simulink model "Stewart_simple"  (R2014a)
settings: Solver=ode3  SolverMode=SingleTasking  StartTime=0.0  StopTime=inf  RelTol=1e-3
libraries: arduinolib x18, neural x6, simulink x1
settings Model: SimulationMode=external  CovModelRefEnable=off  CovSFcnEnable=on  ExtModeTrigDuration=2  Creator=costa  LastModifiedBy=rcostado
settings OptimizationCC: OptimizeModelRefInitCode=on  LifeSpan=1
settings DebuggingCC: UnderspecifiedInitializationDetection=Classic  SolverPrmCheckMsg=none
settings HardwareCC: ProdBitPerInt=16  ProdBitPerPointer=8  ProdIntDivRoundTo=Zero  ProdEndianess=LittleEndian  ProdWordSize=8  ProdHWDeviceType=Atmel->AVR
settings RTWCC: SystemTargetFile=realtime.tlc  GenerateMakefile=off  TemplateMakefile=realtime.tmf  Description=Run on Target Hardware  RTWVerbose=off  ProcessScript=realtime_make_rtw_hook
settings STFCustomTargetCC: TargetLibSuffix=.a  GenerateSampleERTMain=on  ConcurrentExecutionCompliant=off  GeneratePreprocessorConditionals=Use local settings  ERTCustomFileBanners=on  SupportNonInlinedSFcns=off  SupportVariableSizeSignals=on  MATLABClassNameForMDSCustomization=Simulink.SoftwareTarget.ERTCustomization  GRTInterface=off  SystemTargetFile=realtime.tlc
settings ERTTargetCC: CombineOutputUpdateFcns=off  SupportContinuousTime=on  SupportVariableSizeSignals=on  ExtModeTransport=3  ExtModeMexFile=ext_serial_win32_comm  ExtModeMexArgs=0 1 9600  ERTSrcFileBannerTemplate=realtime_code_template.cgt  ERTHdrFileBannerTemplate=realtime_code_template.cgt  ERTDataSrcFileTemplate=realtime_code_template.cgt  ERTDataHdrFileTemplate=realtime_code_template.cgt  ERTCustomFileTemplate=realtime_file_process.tlc

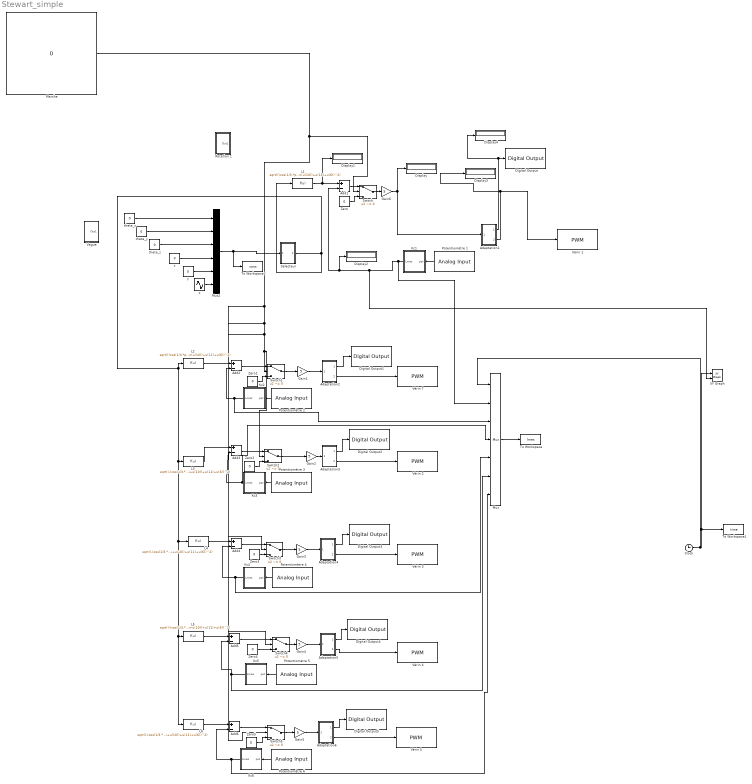
== system Stewart_simple ==
  Adaptation1 : Subsystem
  Adaptation2 : Subsystem
  Adaptation3 : Subsystem
  Adaptation4 : Subsystem
  Adaptation5 : Subsystem
  Adaptation6 : Subsystem
  Add{1..6} (6 alike) : Sum  Inputs=+-
  Clock : Clock
  Digital Output : arduinolib/Digital Output  pinNumber=11
  Digital Output1 : arduinolib/Digital Output  pinNumber=5
  Digital Output2 : arduinolib/Digital Output  pinNumber=3
  Digital Output3 : arduinolib/Digital Output  pinNumber=9
  Digital Output4 : arduinolib/Digital Output  pinNumber=7
  Digital Output5 : arduinolib/Digital Output  pinNumber=13
  Display{,1..4} (5 alike) : Display
  Gain{1..6} (6 alike) : Gain  Gain=5
  Kc1 : Subsystem
  Kc2 : Subsystem
  Kc3 : Subsystem
  Kc4 : Subsystem
  Kc5 : Subsystem
  Kc6 : Subsystem
  L1 : Fcn  Expr=sqrt(((cos(1/3.*pi+u(3))*cos(u(2))-sin(1/3.*pi+u(3))*sin(u(1))*sin(u(2)))*u(7)*cos(u(10))+sin(1/3.*pi+u(3))*cos(u(1))*u(7)*sin(u(10))-u(8)*cos(u(9))+u(4))^2+ ((sin(1/3.*pi+u(3))*cos(u(2))+cos(1/3.*pi+u(3))*sin(u(1))*sin(u(2)))*u(7)*cos(u(10))-cos(1/3.*pi+u(3))*cos(u(1))*u(7)*sin(u(10))-u(8)*sin(u(9))+u(5))^2+ (-cos(u(1))*sin(u(2))*u(7)*cos(u(10))-sin(u(1))*u(7)*sin(u(10))+u(11)+u(6))^2)
  L2 : Fcn  Expr=sqrt(((cos(1/3.*pi+u(3))*cos(u(2))-sin(1/3.*pi+u(3))*sin(u(1))*sin(u(2)))*u(7)*cos(u(10))-sin(1/3.*pi+u(3))*cos(u(1))*u(7)*sin(u(10))+u(8)*cos(1/3.*pi+u(9))+u(4))^2+ ((sin(1/3.*pi+u(3))*cos(u(2))+cos(1/3.*pi+u(3))*sin(u(1))*sin(u(2)))*u(7)*cos(u(10))+cos(1/3.*pi+u(3))*cos(u(1))*u(7)*sin(u(10))-u(8)*sin(1/3.*pi+u(9))+u(5))^2+ (-cos(u(1))*sin(u(2))*u(7)*cos(u(10))+sin(u(1))*u(7)*sin(u(10))+u(11)+u(6))^2)
  L3 : Fcn  Expr=sqrt((-(cos(1/3.*pi+u(3))*cos(u(2))-sin(1/3.*pi+u(3))*sin(u(1))*sin(u(2)))*u(7)*cos(1/3.*pi+u(10))-sin(1/3.*pi+u(3))*cos(u(1))*u(7)*sin(1/3.*pi+u(10))+u(8)*sin(1/6.*pi+u(9))+u(4))^2+(-(sin(1/3.*pi+u(3))*cos(u(2))+cos(1/3.*pi+u(3))*sin(u(1))*sin(u(2)))*u(7)*cos(1/3.*pi+u(10))+cos(1/3.*pi+u(3))*cos(u(1))*u(7)*sin(1/3.*pi+u(10))-u(8)*cos(1/6.*pi+u(9))+u(5))^2+(cos(u(1))*sin(u(2))*u(7)*cos(1/3.*pi+u(10))+sin(u(1))*u(7)*sin(1/3.*pi+u(10))+u(11)+u(6))^2)
  L4 : Fcn  Expr=sqrt((-(cos(1/3.*pi+u(3))*cos(u(2))-sin(1/3.*pi+u(3))*sin(u(1))*sin(u(2)))*u(7)*sin(1/6.*pi+u(10))-sin(1/3.*pi+u(3))*cos(u(1))*u(7)*cos(1/6.*pi+u(10))+u(8)*sin(1/6.*pi+u(9))+u(4))^2+(-(sin(1/3.*pi+u(3))*cos(u(2))+cos(1/3.*pi+u(3))*sin(u(1))*sin(u(2)))*u(7)*sin(1/6.*pi+u(10))+cos(1/3.*pi+u(3))*cos(u(1))*u(7)*cos(1/6.*pi+u(10))+u(8)*cos(1/6.*pi+u(9))+u(5))^2+(cos(u(1))*sin(u(2))*u(7)*sin(1/6.*pi+u(10))+sin(u(1))*u(7)*cos(1/6.*pi+u(10))+u(11)+u(6))^2)
  L5 : Fcn  Expr=sqrt((-(cos(1/3.*pi+u(3))*cos(u(2))-sin(1/3.*pi+u(3))*sin(u(1))*sin(u(2)))*u(7)*sin(1/6.*pi+u(10))+sin(1/3.*pi+u(3))*cos(u(1))*u(7)*cos(1/6.*pi+u(10))+u(8)*cos(1/3.*pi+u(9))+u(4))^2+(-(sin(1/3.*pi+u(3))*cos(u(2))+cos(1/3.*pi+u(3))*sin(u(1))*sin(u(2)))*u(7)*sin(1/6.*pi+u(10))-cos(1/3.*pi+u(3))*cos(u(1))*u(7)*cos(1/6.*pi+u(10))+u(8)*sin(1/3.*pi+u(9))+u(5))^2+(cos(u(1))*sin(u(2))*u(7)*sin(1/6.*pi+u(10))-sin(u(1))*u(7)*cos(1/6.*pi+u(10))+u(11)+u(6))^2)
  L6 : Fcn  Expr=sqrt((-(cos(1/3.*pi+u(3))*cos(u(2))-sin(1/3.*pi+u(3))*sin(u(1))*sin(u(2)))*u(7)*cos(1/3.*pi+u(10))+sin(1/3.*pi+u(3))*cos(u(1))*u(7)*sin(1/3.*pi+u(10))-u(8)*cos(u(9))+u(4))^2+(-(sin(1/3.*pi+u(3))*cos(u(2))+cos(1/3.*pi+u(3))*sin(u(1))*sin(u(2)))*u(7)*cos(1/3.*pi+u(10))-cos(1/3.*pi+u(3))*cos(u(1))*u(7)*sin(1/3.*pi+u(10))+u(8)*sin(u(9))+u(5))^2+(cos(u(1))*sin(u(2))*u(7)*cos(1/3.*pi+u(10))-sin(u(1))*u(7)*sin(1/3.*pi+u(10))+u(11)+u(6))^2)
  Marche : Constant  Value=0
  Mux : Mux  Inputs=7
  Mux2 : Mux  Inputs=6
  Potentiomètre 1 : arduinolib/Analog Input  pinNumber=2  sampleTime=0.001
  Potentiomètre 2 : arduinolib/Analog Input  pinNumber=1  sampleTime=0.001
  Potentiomètre 3 : arduinolib/Analog Input  pinNumber=0  sampleTime=0.001
  Potentiomètre 4 : arduinolib/Analog Input  pinNumber=5  sampleTime=0.001
  Potentiomètre 5 : arduinolib/Analog Input  pinNumber=4  sampleTime=0.001
  Potentiomètre 6 : arduinolib/Analog Input  pinNumber=3  sampleTime=0.001
  Rotation z : Subsystem
  Selecteur : Subsystem
  Switch{,1..5} (6 alike) : Switch  Criteria=u2 ~= 0
  To Workspace : ToWorkspace  VariableName=lmes  SampleTime=-1
  To Workspace1 : ToWorkspace  VariableName=time  SampleTime=-1
  To Workspace2 : ToWorkspace  VariableName=cons  SampleTime=-1
  Vague : Subsystem
  Vérin 1 : arduinolib/PWM  pinNumber=10
  Vérin 2 : arduinolib/PWM  pinNumber=2
  Vérin 3 : arduinolib/PWM  pinNumber=8
  Vérin 4 : arduinolib/PWM  pinNumber=6
  Vérin 5 : arduinolib/PWM  pinNumber=12
  Vérin 7 : arduinolib/PWM  pinNumber=4
  XY Graph : simulink/Sinks/XY Graph  xmin=0  xmax=10  ymin=300  ymax=600  st=-1
  Zero{,1..5} (6 alike) : Constant  Value=0
  theta_x : Constant  Value=0
  theta_y : Constant  Value=0
  theta_z : Constant  Value=0
  x : Constant  Value=0
  y : Constant  Value=0
  z : Sin  Amplitude=50  Frequency=60  SampleTime=0
  wires:
  Potentiomètre 1/1 -> Kc1/1(pot)
  L1/1 -> Display1/1, Add1/1
  Gain6/1 -> Display/1, Adaptation1/1(ecart)
  Adaptation1/1(sens) -> Display4/1, Digital Output/1
  Adaptation1/2(pwm) -> Display3/1, Vérin 1/1
  Selecteur/1(Out1) -> L6/1, L5/1, L4/1, L3/1, L2/1, L1/1
  Mux2/1 -> To Workspace2/1, Selecteur/1(In2)
  Gain1/1 -> Adaptation2/1(ecart)
  L2/1 -> Add2/1
  Adaptation2/1(sens) -> Digital Output1/1
  Adaptation2/2(pwm) -> Vérin 7/1
  Potentiomètre 2/1 -> Kc2/1(pot)
  Kc2/1(Lmes) -> Mux/3, Add2/2
  L3/1 -> Add3/1
  Adaptation3/1(sens) -> Digital Output2/1
  Adaptation3/2(pwm) -> Vérin 2/1
  Gain2/1 -> Adaptation3/1(ecart)
  Potentiomètre 3/1 -> Kc3/1(pot)
  L4/1 -> Add4/1
  Gain3/1 -> Adaptation4/1(ecart)
  Adaptation4/1(sens) -> Digital Output3/1
  Adaptation4/2(pwm) -> Vérin 3/1
  Kc4/1(Lmes) -> Mux/5, Add4/2
  Potentiomètre 4/1 -> Kc4/1(pot)
  L5/1 -> Add5/1
  Adaptation5/1(sens1) -> Digital Output4/1
  Adaptation5/2(pwm1) -> Vérin 4/1
  Potentiomètre 5/1 -> Kc5/1(pot)
  Kc5/1(Lmes) -> Mux/6, Add5/2
  Gain4/1 -> Adaptation5/1(ecart1)
  L6/1 -> Add6/1
  Adaptation6/1(sens) -> Digital Output5/1
  Adaptation6/2(pwm) -> Vérin 5/1
  Potentiomètre 6/1 -> Kc6/1(pot)
  Kc6/1(Lmes) -> Mux/7, Add6/2
  Gain5/1 -> Adaptation6/1(ecart)
  Kc1/1(Lmes) -> Mux/2, XY Graph/2, Display2/1, Add1/2
  Kc3/1(Lmes) -> Mux/4, Add3/2
  z/1 -> Mux2/6
  x/1 -> Mux2/4
  theta_x/1 -> Mux2/1
  y/1 -> Mux2/5
  theta_z/1 -> Mux2/3
  theta_y/1 -> Mux2/2
  Switch/1 -> Gain6/1
  Add1/1 -> Switch/1
  Zero/1 -> Switch/3
  Marche/1 -> Switch5/2, Switch3/2, Switch4/2, Switch2/2, Switch1/2, Switch/2
  Add2/1 -> Switch1/1
  Switch1/1 -> Gain1/1
  Zero1/1 -> Switch1/3
  Switch2/1 -> Gain2/1
  Zero2/1 -> Switch2/3
  Zero3/1 -> Switch3/3
  Switch3/1 -> Gain3/1
  Add4/1 -> Switch3/1
  Switch4/1 -> Gain4/1
  Add5/1 -> Switch4/1
  Zero4/1 -> Switch4/3
  Switch5/1 -> Gain5/1
  Zero5/1 -> Switch5/3
  Add6/1 -> Switch5/1
  Add3/1 -> Switch2/1
  Mux/1 -> To Workspace/1
  Clock/1 -> Mux/1, To Workspace1/1, XY Graph/1

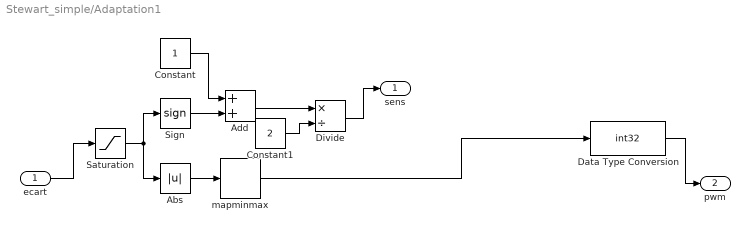
== system Stewart_simple/Adaptation1 ==
  ecart : Inport
  Abs : Abs
  Add : Sum
  Constant : Constant
  Constant1 : Constant  Value=2
  Data Type Conversion : DataTypeConversion  OutDataTypeStr=int32
  Divide : Product  Inputs=*/
  Saturation : Saturate  UpperLimit=200  LowerLimit=-200
  Sign : Signum
  mapminmax : neural/Processing Functions/mapminmax  xmin=0  xmax=200  ymin=1  ymax=255
  sens : Outport
  pwm : Outport  Port=2
  wires:
  ecart/1 -> Saturation/1
  Abs/1 -> mapminmax/1
  Saturation/1 -> Sign/1, Abs/1
  Sign/1 -> Add/2
  Constant/1 -> Add/1
  Add/1 -> Divide/1
  Constant1/1 -> Divide/2
  Divide/1 -> sens/1
  Data Type Conversion/1 -> pwm/1
  mapminmax/1 -> Data Type Conversion/1

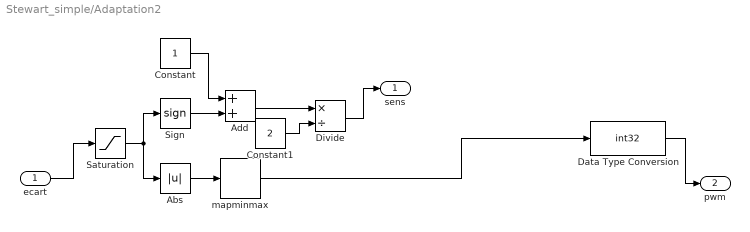
== system Stewart_simple/Adaptation2 ==
  ecart : Inport
  Abs : Abs
  Add : Sum
  Constant : Constant
  Constant1 : Constant  Value=2
  Data Type Conversion : DataTypeConversion  OutDataTypeStr=int32
  Divide : Product  Inputs=*/
  Saturation : Saturate  UpperLimit=200  LowerLimit=-200
  Sign : Signum
  mapminmax : neural/Processing Functions/mapminmax  xmin=0  xmax=200  ymin=1  ymax=255
  sens : Outport
  pwm : Outport  Port=2
  wires:
  ecart/1 -> Saturation/1
  Abs/1 -> mapminmax/1
  Saturation/1 -> Sign/1, Abs/1
  Sign/1 -> Add/2
  Constant/1 -> Add/1
  Add/1 -> Divide/1
  Constant1/1 -> Divide/2
  Divide/1 -> sens/1
  Data Type Conversion/1 -> pwm/1
  mapminmax/1 -> Data Type Conversion/1

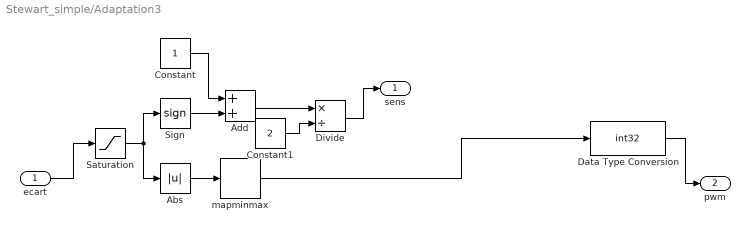
== system Stewart_simple/Adaptation3 ==
  ecart : Inport
  Abs : Abs
  Add : Sum
  Constant : Constant
  Constant1 : Constant  Value=2
  Data Type Conversion : DataTypeConversion  OutDataTypeStr=int32
  Divide : Product  Inputs=*/
  Saturation : Saturate  UpperLimit=200  LowerLimit=-200
  Sign : Signum
  mapminmax : neural/Processing Functions/mapminmax  xmin=0  xmax=200  ymin=1  ymax=255
  sens : Outport
  pwm : Outport  Port=2
  wires:
  ecart/1 -> Saturation/1
  Abs/1 -> mapminmax/1
  Saturation/1 -> Sign/1, Abs/1
  Sign/1 -> Add/2
  Constant/1 -> Add/1
  Add/1 -> Divide/1
  Constant1/1 -> Divide/2
  Divide/1 -> sens/1
  Data Type Conversion/1 -> pwm/1
  mapminmax/1 -> Data Type Conversion/1

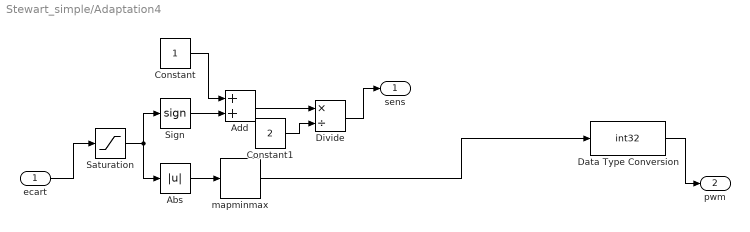
== system Stewart_simple/Adaptation4 ==
  ecart : Inport
  Abs : Abs
  Add : Sum
  Constant : Constant
  Constant1 : Constant  Value=2
  Data Type Conversion : DataTypeConversion  OutDataTypeStr=int32
  Divide : Product  Inputs=*/
  Saturation : Saturate  UpperLimit=200  LowerLimit=-200
  Sign : Signum
  mapminmax : neural/Processing Functions/mapminmax  xmin=0  xmax=200  ymin=1  ymax=255
  sens : Outport
  pwm : Outport  Port=2
  wires:
  ecart/1 -> Saturation/1
  Abs/1 -> mapminmax/1
  Saturation/1 -> Sign/1, Abs/1
  Sign/1 -> Add/2
  Constant/1 -> Add/1
  Add/1 -> Divide/1
  Constant1/1 -> Divide/2
  Divide/1 -> sens/1
  Data Type Conversion/1 -> pwm/1
  mapminmax/1 -> Data Type Conversion/1

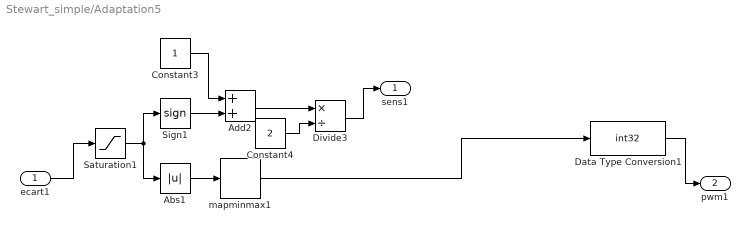
== system Stewart_simple/Adaptation5 ==
  ecart1 : Inport
  Abs1 : Abs
  Add2 : Sum
  Constant3 : Constant
  Constant4 : Constant  Value=2
  Data Type Conversion1 : DataTypeConversion  OutDataTypeStr=int32
  Divide3 : Product  Inputs=*/
  Saturation1 : Saturate  UpperLimit=200  LowerLimit=-200
  Sign1 : Signum
  mapminmax1 : neural/Processing Functions/mapminmax  xmin=0  xmax=200  ymin=1  ymax=255
  sens1 : Outport
  pwm1 : Outport  Port=2
  wires:
  ecart1/1 -> Saturation1/1
  Abs1/1 -> mapminmax1/1
  Saturation1/1 -> Sign1/1, Abs1/1
  Sign1/1 -> Add2/2
  Constant3/1 -> Add2/1
  Add2/1 -> Divide3/1
  Constant4/1 -> Divide3/2
  Divide3/1 -> sens1/1
  Data Type Conversion1/1 -> pwm1/1
  mapminmax1/1 -> Data Type Conversion1/1

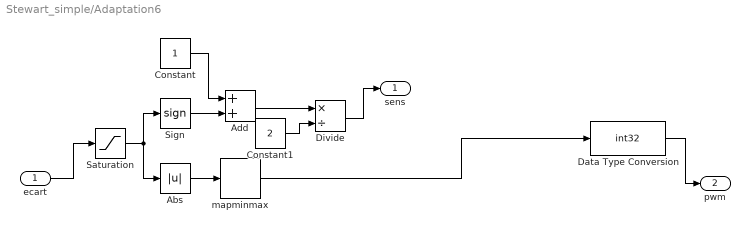
== system Stewart_simple/Adaptation6 ==
  ecart : Inport
  Abs : Abs
  Add : Sum
  Constant : Constant
  Constant1 : Constant  Value=2
  Data Type Conversion : DataTypeConversion  OutDataTypeStr=int32
  Divide : Product  Inputs=*/
  Saturation : Saturate  UpperLimit=200  LowerLimit=-200
  Sign : Signum
  mapminmax : neural/Processing Functions/mapminmax  xmin=0  xmax=200  ymin=1  ymax=255
  sens : Outport
  pwm : Outport  Port=2
  wires:
  ecart/1 -> Saturation/1
  Abs/1 -> mapminmax/1
  Saturation/1 -> Sign/1, Abs/1
  Sign/1 -> Add/2
  Constant/1 -> Add/1
  Add/1 -> Divide/1
  Constant1/1 -> Divide/2
  Divide/1 -> sens/1
  Data Type Conversion/1 -> pwm/1
  mapminmax/1 -> Data Type Conversion/1

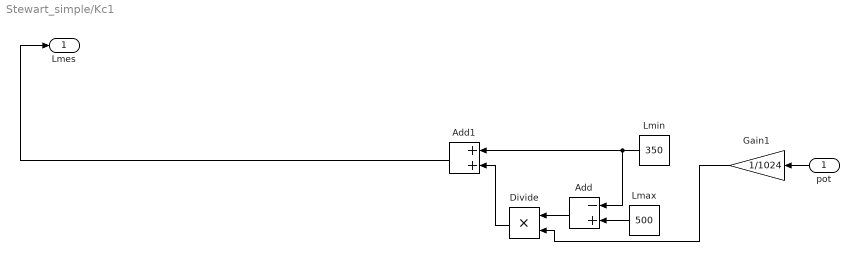
== system Stewart_simple/Kc1 ==
  pot : Inport
  Add : Sum  Inputs=-+
  Add1 : Sum
  Divide : Product  Inputs=**
  Gain1 : Gain  Gain=1/1024
  Lmax : Constant  Value=500
  Lmin : Constant  Value=350
  Lmes : Outport
  wires:
  Lmin/1 -> Add1/1, Add/1
  Lmax/1 -> Add/2
  Gain1/1 -> Divide/2
  Divide/1 -> Add1/2
  Add1/1 -> Lmes/1
  pot/1 -> Gain1/1
  Add/1 -> Divide/1

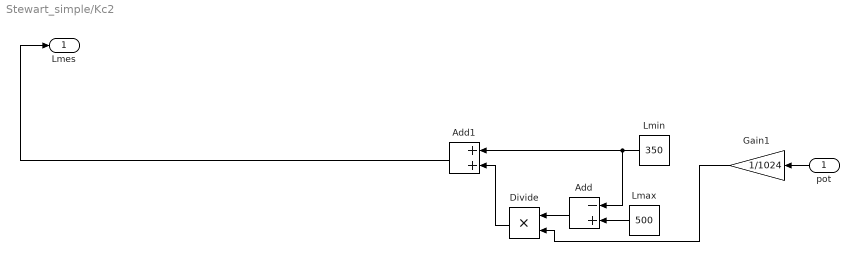
== system Stewart_simple/Kc2 ==
  pot : Inport
  Add : Sum  Inputs=-+
  Add1 : Sum
  Divide : Product  Inputs=**
  Gain1 : Gain  Gain=1/1024
  Lmax : Constant  Value=500
  Lmin : Constant  Value=350
  Lmes : Outport
  wires:
  Lmin/1 -> Add1/1, Add/1
  Lmax/1 -> Add/2
  Gain1/1 -> Divide/2
  Divide/1 -> Add1/2
  Add1/1 -> Lmes/1
  pot/1 -> Gain1/1
  Add/1 -> Divide/1

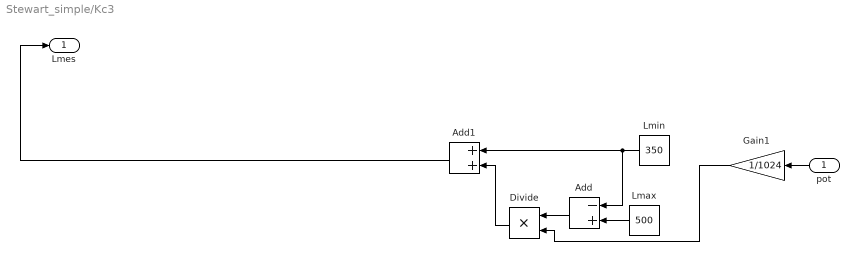
== system Stewart_simple/Kc3 ==
  pot : Inport
  Add : Sum  Inputs=-+
  Add1 : Sum
  Divide : Product  Inputs=**
  Gain1 : Gain  Gain=1/1024
  Lmax : Constant  Value=500
  Lmin : Constant  Value=350
  Lmes : Outport
  wires:
  Lmin/1 -> Add1/1, Add/1
  Lmax/1 -> Add/2
  Gain1/1 -> Divide/2
  Divide/1 -> Add1/2
  Add1/1 -> Lmes/1
  pot/1 -> Gain1/1
  Add/1 -> Divide/1

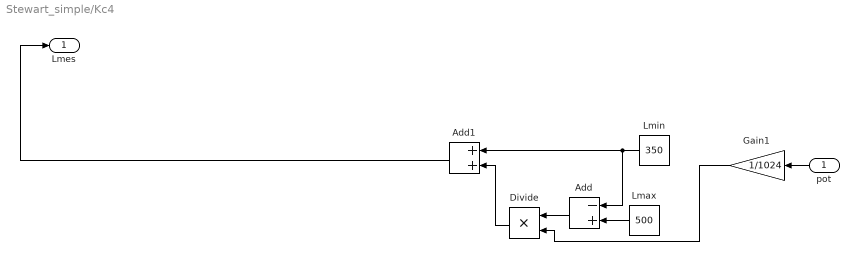
== system Stewart_simple/Kc4 ==
  pot : Inport
  Add : Sum  Inputs=-+
  Add1 : Sum
  Divide : Product  Inputs=**
  Gain1 : Gain  Gain=1/1024
  Lmax : Constant  Value=500
  Lmin : Constant  Value=350
  Lmes : Outport
  wires:
  Lmin/1 -> Add1/1, Add/1
  Lmax/1 -> Add/2
  Gain1/1 -> Divide/2
  Divide/1 -> Add1/2
  Add1/1 -> Lmes/1
  pot/1 -> Gain1/1
  Add/1 -> Divide/1

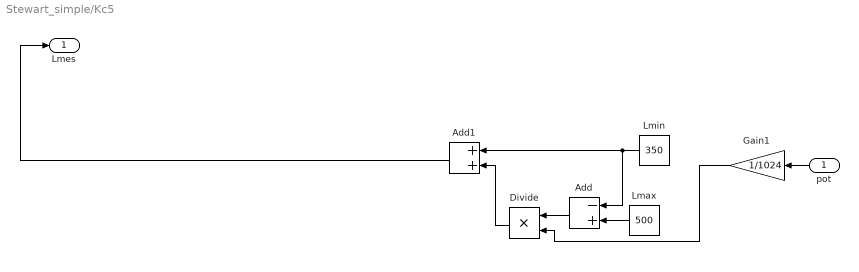
== system Stewart_simple/Kc5 ==
  pot : Inport
  Add : Sum  Inputs=-+
  Add1 : Sum
  Divide : Product  Inputs=**
  Gain1 : Gain  Gain=1/1024
  Lmax : Constant  Value=500
  Lmin : Constant  Value=350
  Lmes : Outport
  wires:
  Lmin/1 -> Add1/1, Add/1
  Lmax/1 -> Add/2
  Gain1/1 -> Divide/2
  Divide/1 -> Add1/2
  Add1/1 -> Lmes/1
  pot/1 -> Gain1/1
  Add/1 -> Divide/1

== system Stewart_simple/Kc6 ==
  pot : Inport
  Add : Sum  Inputs=-+
  Add1 : Sum
  Divide : Product  Inputs=**
  Gain1 : Gain  Gain=1/1024
  Lmax : Constant  Value=500
  Lmin : Constant  Value=350
  Lmes : Outport
  wires:
  Lmin/1 -> Add1/1, Add/1
  Lmax/1 -> Add/2
  Gain1/1 -> Divide/2
  Divide/1 -> Add1/2
  Add1/1 -> Lmes/1
  pot/1 -> Gain1/1
  Add/1 -> Divide/1

== system Stewart_simple/Rotation z ==
  Mux1 : Mux  Inputs=6
  theta_x : Constant  Value=0
  theta_y : Constant  Value=0
  theta_z : Sin  Amplitude=pi/8  Frequency=40  SampleTime=0
  x : Constant  Value=0
  y : Constant  Value=0
  z : Constant  Value=0
  Out1 : Outport
  wires:
  theta_y/1 -> Mux1/2
  theta_z/1 -> Mux1/3
  y/1 -> Mux1/5
  theta_x/1 -> Mux1/1
  x/1 -> Mux1/4
  z/1 -> Mux1/6
  Mux1/1 -> Out1/1

== system Stewart_simple/Selecteur ==
  In2 : Inport
  Mux : Mux  Inputs=2
  Paramètres mécanisme : Subsystem
  Out1 : Outport
  wires:
  Paramètres mécanisme/1(Out1) -> Mux/2
  In2/1 -> Mux/1
  Mux/1 -> Out1/1

== system Stewart_simple/Vague ==
  Mux1 : Mux  Inputs=6
  theta_x : Sin  Amplitude=pi/8  Frequency=40  SampleTime=0
  theta_y : Sin  Amplitude=pi/8  Frequency=40  Phase=pi/2  SampleTime=0
  theta_z : Constant  Value=0
  x : Constant  Value=0
  y : Constant  Value=0
  z : Constant  Value=0
  Out1 : Outport
  wires:
  theta_y/1 -> Mux1/2
  theta_z/1 -> Mux1/3
  y/1 -> Mux1/5
  theta_x/1 -> Mux1/1
  x/1 -> Mux1/4
  z/1 -> Mux1/6
  Mux1/1 -> Out1/1

== system Stewart_simple/Selecteur/Paramètres mécanisme ==
  Mux1 : Mux  Inputs=5
  alpha : Constant  Value=0.007
  beta : Constant  Value=0.009
  h : Constant  Value=380
  rf : Constant  Value=270
  rm : Constant  Value=200
  Out1 : Outport
  wires:
  Mux1/1 -> Out1/1
  rm/1 -> Mux1/1
  rf/1 -> Mux1/2
  alpha/1 -> Mux1/3
  beta/1 -> Mux1/4
  h/1 -> Mux1/5
